simulink model "Vehicle_Speed_sim"  (R2026a)
settings: Solver=VariableStepAuto
InitFcn:
  | vehicle_speed_params_init
values from neighbouring files (symbols this model uses):
  Aero_Cd_A_m2 = Simulink.Parameter(1.2)    [vehicle_speed_params_init.m]
  Air_Density_kgm3 = Simulink.Parameter(1.225)    [vehicle_speed_params_init.m]
  Brake_Force_N = Simulink.Parameter(40000)    [vehicle_speed_params_init.m]
  Gravity_ms2 = Simulink.Parameter(9.81)    [vehicle_speed_params_init.m]
  Rolling_Resist_Coeff = Simulink.Parameter(0.015)    [vehicle_speed_params_init.m]
  Vehicle_Mass_kg = Simulink.Parameter(798)    [vehicle_speed_params_init.m]
  Vehicle_Speed_Init = Simulink.Parameter(100)    [vehicle_speed_params_init.m]
  Wheel_Radius_m = Simulink.Parameter(0.33)    [vehicle_speed_params_init.m]
settings Model: Creator=nixiaofeng  LastModifiedBy=nixiaofeng

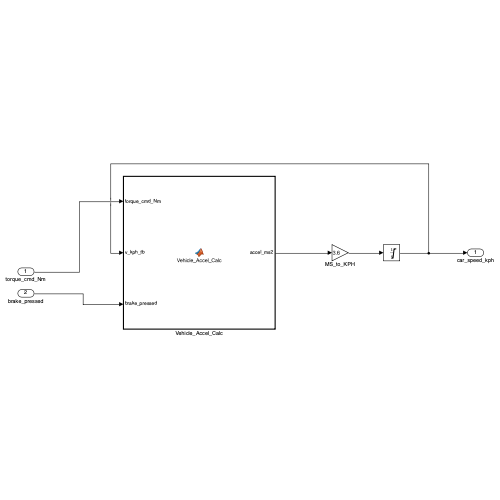
[thumbnail: Simulink's stored preview of the top-level diagram]
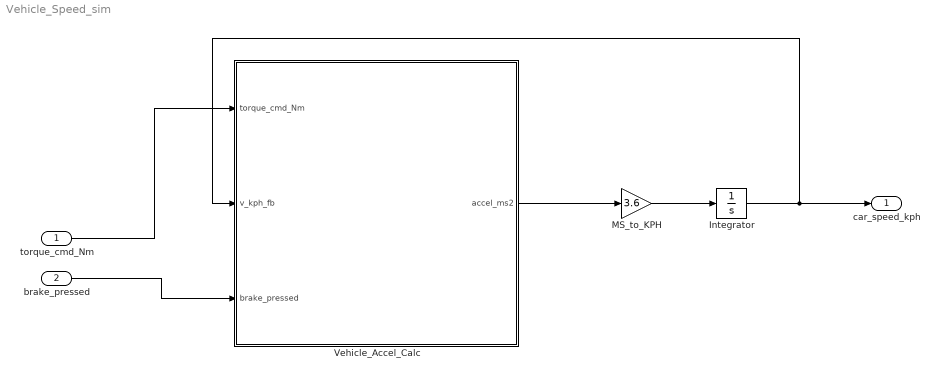
== system Vehicle_Speed_sim ==
  torque_cmd_Nm : Inport
  brake_pressed : Inport  Port=2
  Integrator : Integrator  InitialCondition=Vehicle_Speed_Init  LimitOutput=on  LowerSaturationLimit=0
  MS_to_KPH : Gain  Gain=3.6
  Vehicle_Accel_Calc : MATLAB Function  TreatAsAtomicUnit=on
  car_speed_kph : Outport
  wires:
  torque_cmd_Nm/1 -> Vehicle_Accel_Calc/1(torque_cmd_Nm)
  brake_pressed/1 -> Vehicle_Accel_Calc/3(brake_pressed)
  Vehicle_Accel_Calc/1(accel_ms2) -> MS_to_KPH/1
  MS_to_KPH/1 -> Integrator/1
  Integrator/1 -> Vehicle_Accel_Calc/2(v_kph_fb), car_speed_kph/1

== matlab function Vehicle_Speed_sim/Vehicle_Accel_Calc ==
  data: torque_cmd_Nm input; accel_ms2 output; v_kph_fb input; brake_pressed input; Wheel_Radius_m parameter; Air_Density_kgm3 parameter; Rolling_Resist_Coeff parameter; Brake_Force_N parameter; Aero_Cd_A_m2 parameter; Vehicle_Mass_kg parameter; Gravity_ms2 parameter
function accel_ms2 = Vehicle_Accel_Calc(torque_cmd_Nm, v_kph_fb, brake_pressed, Wheel_Radius_m, Air_Density_kgm3, Rolling_Resist_Coeff, Brake_Force_N, Aero_Cd_A_m2, Vehicle_Mass_kg, Gravity_ms2)
v_ms = v_kph_fb / 3.6;
F_drive = torque_cmd_Nm / Wheel_Radius_m;
F_drag = 0.5 * Air_Density_kgm3 * Aero_Cd_A_m2 * v_ms^2;
F_roll = Rolling_Resist_Coeff * Vehicle_Mass_kg * Gravity_ms2;
F_brake = brake_pressed * Brake_Force_N;
F_net = F_drive - F_drag - F_roll - F_brake;
accel_ms2 = F_net / Vehicle_Mass_kg;
end
